simulink model "HLB_LDMCoeffs_cpp"  (R2019b)
settings: Solver=FixedStepDiscrete  StartTime=0.0  StopTime=10.0  FixedStep=0.01  RelTol=1e-3
settings Model: Creator=IGG2BP  LastModifiedBy=IGG2BP
settings ModelReferenceCC: ModelReferenceNumInstancesAllowed=Single

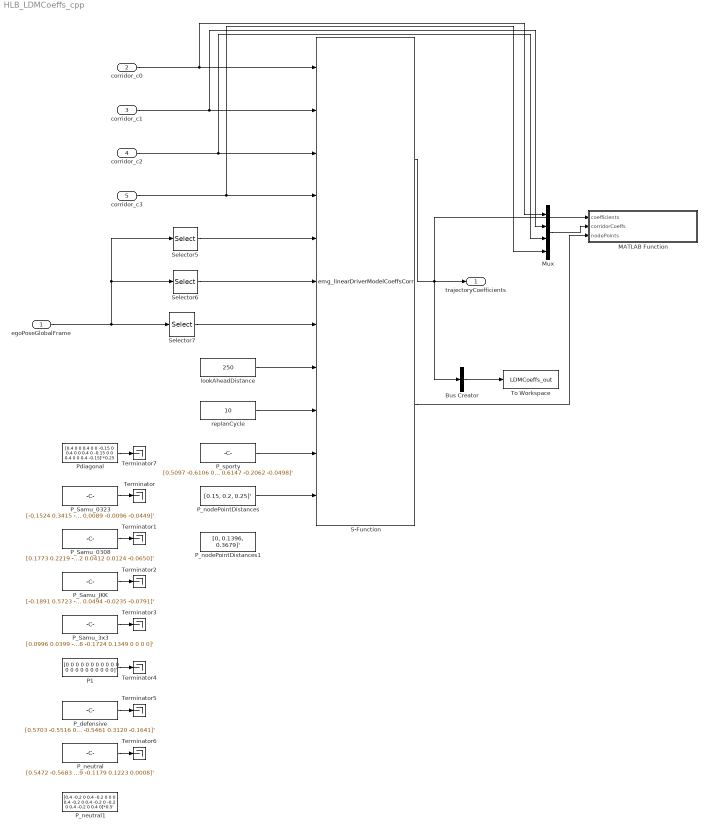
== system HLB_LDMCoeffs_cpp ==
  egoPoseGlobalFrame : Inport
  corridor_c0 : Inport  Port=2
  corridor_c1 : Inport  Port=3
  corridor_c2 : Inport  Port=4
  corridor_c3 : Inport  Port=5
  Bus Creator : BusCreator  Inputs=1
  MATLAB Function : MATLAB Function  TreatAsAtomicUnit=on
  Mux : Mux
  P1 : Constant  Value=[0 0 0 0 0 0 0 0 0 0 0 0 0 0 0 0 0 0 0 0 0]'
  P_Samu_0308 : Constant  Value=[0.1773 0.2219 -0.2682 -0.0332 0.0887 0.0013 0.0761 -0.3368 0.7714 -0.3123 0.0194 -0.0027 0.0293 0.0384 0.2913 -0.4504 0.2953 -0.0362 0.0412 0.0124 -0.0650]'
  P_Samu_0323 : Constant  Value=[-0.1524 0.3415 -0.1253 -0.0464 0.0239 -0.0055 0.0215 0.1143 0.0686 -0.1218 -0.0161 0.0354 0.0297 -0.0039 0.3901 -0.5318 0.2184 0.0146 0.0089 -0.0096 -0.0449]'
  P_Samu_3x3 : Constant  Value=[0.0996 0.0399 -0.0811 0 0 0 0 -0.0754 0.2313 -0.0940 0 0 0 0 0.1228 -0.1724 0.1349 0 0 0 0]'
  P_Samu_JKK : Constant  Value=[-0.1891 0.5723 -0.2526 -0.0105 0.0167 -0.0250 0.0681 -0.4980 0.9711 -0.3461 0.0010 -0.0047 0.0333 0.0391 0.6295 -0.8867 0.3919 0.0183 0.0494 -0.0235 -0.0791]'
  P_defensive : Constant  Value="[0.5703 -0.5516 0.0204 -0.0826 0.2758 -0.1267 -0.1641 -0.0189 0.1369 -0.0802 -0.9290 1.2190  -0.2236 -0.1641 -0.6678 0.8077 -0.1056 0.3043 -0.5461 0.3120 -0.1641]'"
  P_neutral : Constant  Value=[0.5472 -0.5683 0.0506 0.0006 0.1948 -0.1471 0.0008 0.2303 -0.1777 -0.0226 -0.6646 0.9578 -0.2457 0.0008 -0.0388 0.0900 -0.0114 0.0569 -0.1179 0.1223 0.0008]'
  P_neutral1 : Constant  Value=[0.4 -0.2 0 0.4 -0.2 0 0 0 0.4 -0.2 0 0.4 -0.2 0 -0.2 0 0.4 -0.2 0 0.4 0]*0.5'
  P_nodePointDistances : Constant  Value=[0.15, 0.2, 0.25]'
  P_nodePointDistances1 : Constant  Value=[0, 0.1396, 0.3679]'
  P_sporty : Constant  Value=[0.5097 -0.6106 0.1487 0.2415 -0.0941 -0.0935 -0.0498 0.3298 -0.2866 0.0218 0.0035 0.2626 -0.1936 -0.0498 0.019 0.1285 -0.0701 -0.316 0.6147 -0.2062 -0.0498]'
  Pdiagonal : Constant  Value=[0.4 0 0 0.4 0 0 -0.15 0 0.4 0 0 0.4 0 -0.15 0 0 0.4 0 0 0.4 -0.15]'*0.25
  S-Function : S-Function  FunctionName=emg_linearDriverModelCoeffsCorr  SFunctionDeploymentMode=off  EnableBusSupport=off
  Selector5 : Selector  InputPortWidth=3  IndexOptions=Index vector (dialog)  Indices=1  OutputSizes=1
  Selector6 : Selector  InputPortWidth=3  IndexOptions=Index vector (dialog)  Indices=2  OutputSizes=1
  Selector7 : Selector  InputPortWidth=3  IndexOptions=Index vector (dialog)  Indices=3  OutputSizes=1
  Terminator{,1..7} (8 alike) : Terminator
  To Workspace : ToWorkspace  VariableName=LDMCoeffs_out  SaveFormat=Timeseries  SampleTime=-1
  lookAheadDistance : Constant  Value=250
  replanCycle : Constant  Value=10
  trajectoryCoefficients : Outport
  wires:
  Bus Creator/1 -> To Workspace/1
  egoPoseGlobalFrame/1 -> Selector6/1, Selector5/1, Selector7/1
  P_Samu_JKK/1 -> Terminator2/1
  P_Samu_0308/1 -> Terminator1/1
  corridor_c3/1 -> Mux/4, S-Function/4
  P_Samu_0323/1 -> Terminator/1
  corridor_c2/1 -> Mux/3, S-Function/3
  corridor_c1/1 -> Mux/2, S-Function/2
  corridor_c0/1 -> Mux/1, S-Function/1
  P_Samu_3x3/1 -> Terminator3/1
  S-Function/1 -> MATLAB Function/1(coefficients), Bus Creator/1, trajectoryCoefficients/1
  P_defensive/1 -> Terminator5/1
  P_neutral/1 -> Terminator6/1
  Selector5/1 -> S-Function/5
  Selector6/1 -> S-Function/6
  Selector7/1 -> S-Function/7
  lookAheadDistance/1 -> S-Function/8
  replanCycle/1 -> S-Function/9
  Mux/1 -> MATLAB Function/2(corridorCoeffs)
  S-Function/2 -> MATLAB Function/3(nodePoints)
  P_nodePointDistances/1 -> S-Function/11
  P1/1 -> Terminator4/1
  P_sporty/1 -> S-Function/10
  Pdiagonal/1 -> Terminator7/1

== matlab function HLB_LDMCoeffs_cpp/MATLAB Function ==
  data: coefficients input; corridorCoeffs input; nodePoints input
function fcn(coefficients, corridorCoeffs, nodePoints)
figure(1);
x = linspace(0,coefficients(8),50);
x2 = linspace(coefficients(8),coefficients(16),50);
y = coefficients(1) + coefficients(2)*x+ coefficients(3)/2*x.^2 + coefficients(4)/6*x.^3 + coefficients(5)/24*x.^4 + coefficients(6)/120*x.^5;
y_corr = corridorCoeffs(1) + corridorCoeffs(2)*[x x2]+ corridorCoeffs(3)*[x x2].^2 + corridorCoeffs(4)*[x x2].^3;

y2 = coefficients(9) + coefficients(10)*x2+ coefficients(11)/2*x2.^2 + coefficients(12)/6*x2.^3 + coefficients(13)/24*x2.^4 + coefficients(14)/120*x2.^5;
yLeft = y_corr+1.875;
yRight = y_corr-1.875;
plot(x,y, 'k', x2, y2, 'k', [x x2],y_corr, 'b', [x x2],yLeft, 'r--', [x x2],yRight, 'g--', nodePoints(1:2:8), nodePoints(2:2:8), 'bo'); xlim([-5, x(end)]); grid on;
xlim([-5,100]);ylim([-10, 10]);
